simulink model "WithStateMachine_decoderN2"  (R2016b)
settings: Solver=FixedStepDiscrete  StartTime=0.0  StopTime=10.0  RelTol=1e-3
settings Model: DataTypeOverride=Off  Creator=hasee  LastModifiedBy=hasee
settings DataIOCC: LimitDataPoints=on  SaveOutput=off  SaveTime=off
settings OptimizationCC: BlockReduction=off  ConditionallyExecuteInputs=off  DefaultParameterBehavior=Inlined  LifeSpan=inf
settings DebuggingCC: AlgebraicLoopMsg=error  SingleTaskRateTransMsg=error  AllowSymbolicDim=off  StrictBusMsg=ErrorOnBusTreatedAsVector  SFUnexpectedBacktrackingDiag=warning  SFNoUnconditionalDefaultTransitionDiag=warning  SFExecutionAtInitializationDiag=none
settings HardwareCC: ProdBitPerPointer=32  ProdBitPerSizeT=32  ProdBitPerPtrDiffT=32  ProdLargestAtomicFloat=None  ProdIntDivRoundTo=Undefined  ProdEndianess=Unspecified  ProdWordSize=32  ProdHWDeviceType=ASIC/FPGA->ASIC/FPGA  ProdEqTarget=off
settings GRTTargetCC: TargetLangStandard=C89/C90 (ANSI)  GeneratePreprocessorConditionals=Disable all
settings ConfigComp: CovScope=ReferencedModels  CovMetricSettings=dw  CovHtmlReporting=on  CovSaveCumulativeToWorkspaceVar=on  CovSaveSingleToWorkspaceVar=on  CovExternalEMLEnable=off  CovSFcnEnable=off

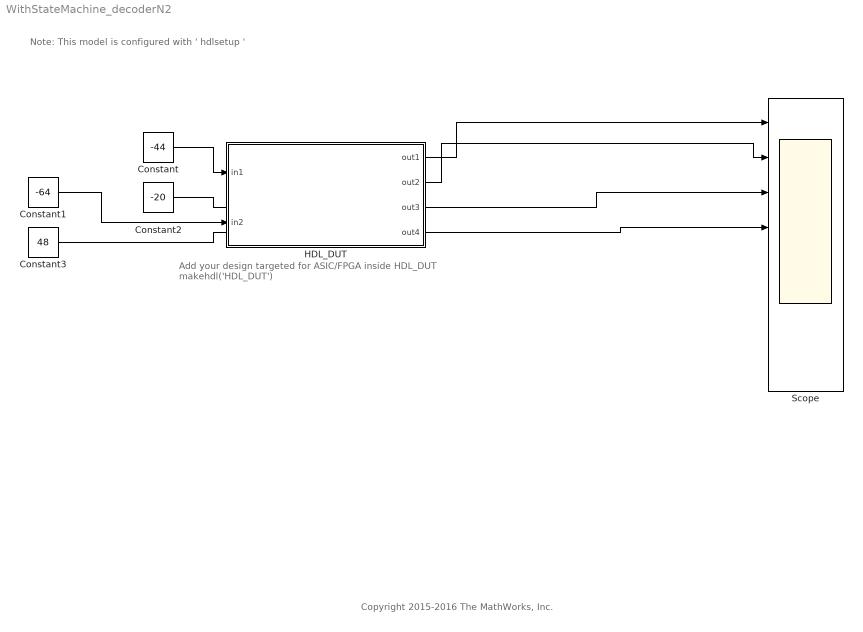
== system WithStateMachine_decoderN2 ==
  note: Note: This model is configured with ' hdlsetup '
  note: Add your design targeted for ASIC/FPGA inside HDL_DUT
      | makehdl('HDL_DUT')
  note: Copyright 2015-2016 The MathWorks, Inc.
  Constant : Constant  Value=-44  OutDataTypeStr=int8  SampleTime=-1
  Constant1 : Constant  Value=-64  OutDataTypeStr=int8  SampleTime=-1
  Constant2 : Constant  Value=-20  OutDataTypeStr=int8  SampleTime=-1
  Constant3 : Constant  Value=48  OutDataTypeStr=int8  SampleTime=-1
  HDL_DUT : Subsystem
  Scope : Scope  NumInputPorts=8
  wires:
  Constant/1 -> HDL_DUT/1(in1)
  Constant1/1 -> HDL_DUT/2(in2)
  HDL_DUT/1(out1) -> Scope/1
  HDL_DUT/2(out2) -> Scope/2
  HDL_DUT/3(out3) -> Scope/3
  Constant2/1 -> ?
  Constant3/1 -> ?
  HDL_DUT/4(out4) -> Scope/4

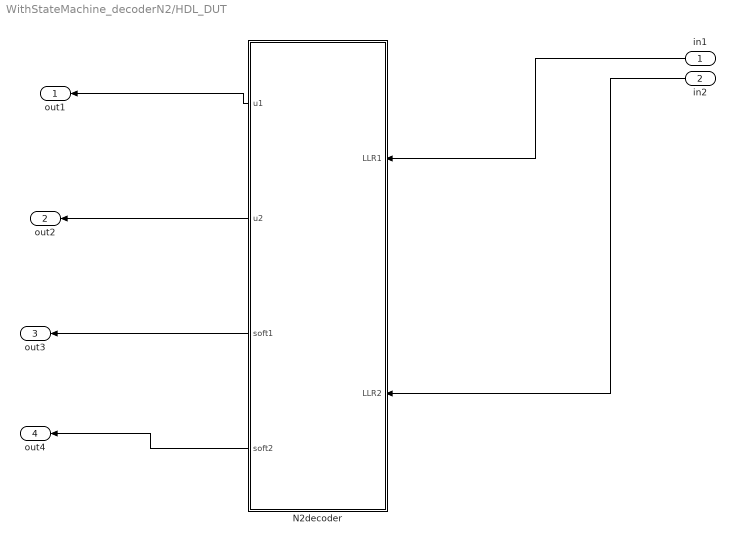
== system WithStateMachine_decoderN2/HDL_DUT ==
  in1 : Inport
  in2 : Inport  Port=2
  N2decoder : MATLAB Function  TreatAsAtomicUnit=on
  out1 : Outport
  out2 : Outport  Port=2
  out3 : Outport  Port=3
  out4 : Outport  Port=4
  wires:
  N2decoder/1(u1) -> out1/1
  N2decoder/2(u2) -> out2/1
  N2decoder/4(soft2) -> out4/1
  N2decoder/3(soft1) -> out3/1
  in1/1 -> N2decoder/1(LLR1)
  in2/1 -> N2decoder/2(LLR2)

== matlab function WithStateMachine_decoderN2/HDL_DUT/N2decoder ==
  data: LLR1 input; u1 output; u2 output; soft1 output; LLR2 input; soft2 output
function [u1,u2,soft1,soft2] = fcn(LLR1,LLR2)
%状态机默认状态是S1（为0）
%每个输出都需要在每一个case里面定义值，或者一开始就定义初值。
%思路：全部状态机操作的都是reg，到最后一个状态的时候统一把所有output都输出reg里面的值，在此之前output可以都为0；
persistent state_reg;
persistent LLR1_reg;
persistent LLR2_reg;
persistent L21y12_reg;
persistent L22y12u11_reg;

persistent u1_reg;
persistent soft1_reg;
persistent u2_reg;
persistent soft2_reg;


if isempty(state_reg)
    state_reg = fi(0, 0, 2, 0, hdlfimath);
    LLR1_reg=  LLR1;
    LLR2_reg=  LLR2;
    %初始化计算u1需要的LLR
    L21y12_reg=int8(0);
    %初始化计算u2需要的LLR
    L22y12u12_reg=int8(0);
    
    %初始化output的寄存器
    u1_reg=false;
    soft1_reg=int8(0);
    u2_reg=false;
    soft2_reg=int8(0);
end

S1 = 0;
S2 = 1;

soft1=soft1_reg;
u1=u1_reg;
soft2=soft2_reg;
u2=u2_reg;
%有限状态机
switch (state_reg)
    case S1
        L21y12_reg=f(LLR1_reg,LLR2_reg);
        soft1_reg=L21y12_reg;
        u1_reg=decide(soft1_reg,1);
        state_reg(1) = S2;
    case S2
        L22y12u12_reg=g(LLR1_reg,LLR2_reg,u1_reg);
        soft2_reg=L22y12u12_reg;
        u2_reg=decide(soft2_reg,2);
end



%判定输出u函数开始；根据软信息和冻结比特位信息；FZlookup是冻结比特位置信息，false代表这一位是冻结比特
function out = decide(soft,position)
persistent FZlookup;
if isempty(FZlookup)
    FZlookup = [false;false;true;true];
end
if FZlookup(position) == true
    if soft > 0  %PCparams.LLR(1) 就是根据最左边的LLR硬裁决
        out = false;
    else
        out = true;
    end
else
    out =FZlookup(position);
end%判定输出u函数结束


function out = f(in1,in2)
%f函数开始
if (in1>0 && in2>0) ||(in1<0 && in2<0)
    out=min(abs(in1),abs(in2));
    %f函数当符号为正时结束
else
    out=-min(abs(in1),abs(in2));
    %f函数当符号为负时结束
end


function out = g(in1,in2,b)
%g函数开始
if (b == 0)
    out=in1 + in2;
    %g函数当b==0时结束
else
    out=-in1 + in2;
    %g函数当b==1时结束
end
